simulink model "equivalence"  (R2021b)
settings: Solver=FixedStepAuto  StartTime=0.0  StopTime=10  FixedStep=0.0001  RelTol=1e-3
settings Model: PauseTimes=0.1  Creator=O  LastModifiedBy=ojiken

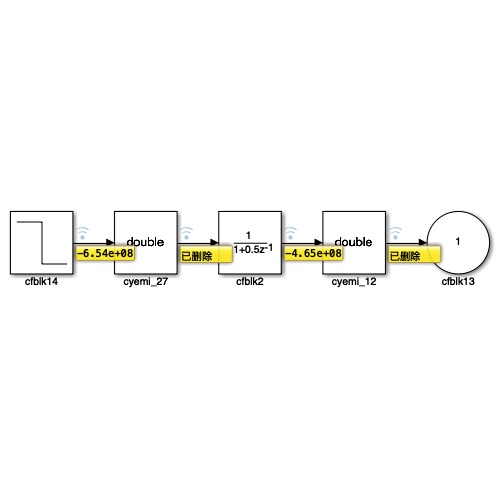
[thumbnail: Simulink's stored preview of the top-level diagram]
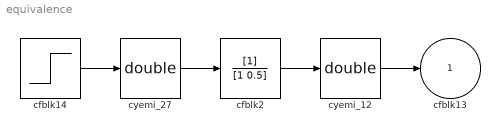
== system equivalence ==
  cfblk14 : Step  Time=[6.000000]  Before=[769690289.111915]  After=[-653636333.758309]  SampleTime=0
  cfblk2 : DiscreteFilter  SampleTime=1
  cyemi_12 : DataTypeConversion  OutDataTypeStr=double
  cyemi_27 : DataTypeConversion  OutDataTypeStr=double
  cfblk13 : Outport
  wires:
  cfblk2/1 -> cyemi_12/1
  cfblk14/1 -> cyemi_27/1
  cyemi_27/1 -> cfblk2/1
  cyemi_12/1 -> cfblk13/1
